simulink model "htx_intent_estimator"  (R2024b)
settings: Solver=VariableStepAuto  StartTime=0.0  StopTime=10.0  RelTol=1e-3
settings Model: Creator=lukec  LastModifiedBy=lukec

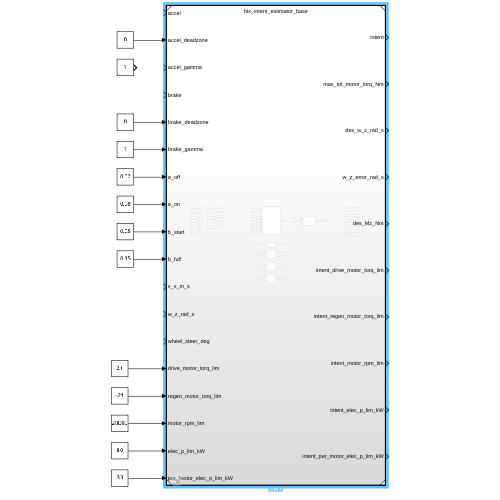
[thumbnail: Simulink's stored preview of the top-level diagram]
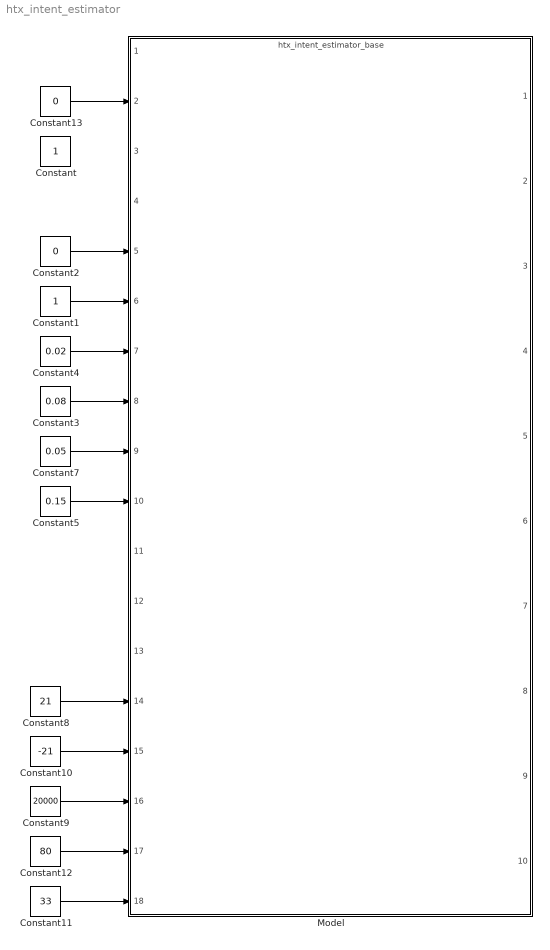
== system htx_intent_estimator ==
  Constant : Constant
  Constant1 : Constant
  Constant10 : Constant  Value=-21
  Constant11 : Constant  Value=33
  Constant12 : Constant  Value=80
  Constant13 : Constant  Value=0
  Constant2 : Constant  Value=0
  Constant3 : Constant  Value=0.08
  Constant4 : Constant  Value=0.02
  Constant5 : Constant  Value=0.15
  Constant7 : Constant  Value=0.05
  Constant8 : Constant  Value=21
  Constant9 : Constant  Value=20000
  Model : ModelReference  ModelNameDialog=htx_intent_estimator_base.slx  SimulationMode=Normal  ModelReferenceVersion=1.6
  wires:
  Constant2/1 -> Model/5
  Constant1/1 -> Model/6
  Constant4/1 -> Model/7
  Constant3/1 -> Model/8
  Constant7/1 -> Model/9
  Constant5/1 -> Model/10
  Constant8/1 -> Model/14
  Constant10/1 -> Model/15
  Constant9/1 -> Model/16
  Constant12/1 -> Model/17
  Constant11/1 -> Model/18
  Constant13/1 -> Model/2
